simulink model "Test_algo_only"  (R2020b)
settings: Solver=ode4  StartTime=0.0  StopTime=0.05  FixedStep=0.001  RelTol=1e-3
values from neighbouring files (symbols this model uses):
  FFT_LENGTH = 256    [Init.m]
  Sampling_rate = 256e3    (= 256000)    [Init.m]
undefined symbols (not defined in the file or in its folder): InvMp, RotX
settings Model: Creator=franc  LastModifiedBy=franc

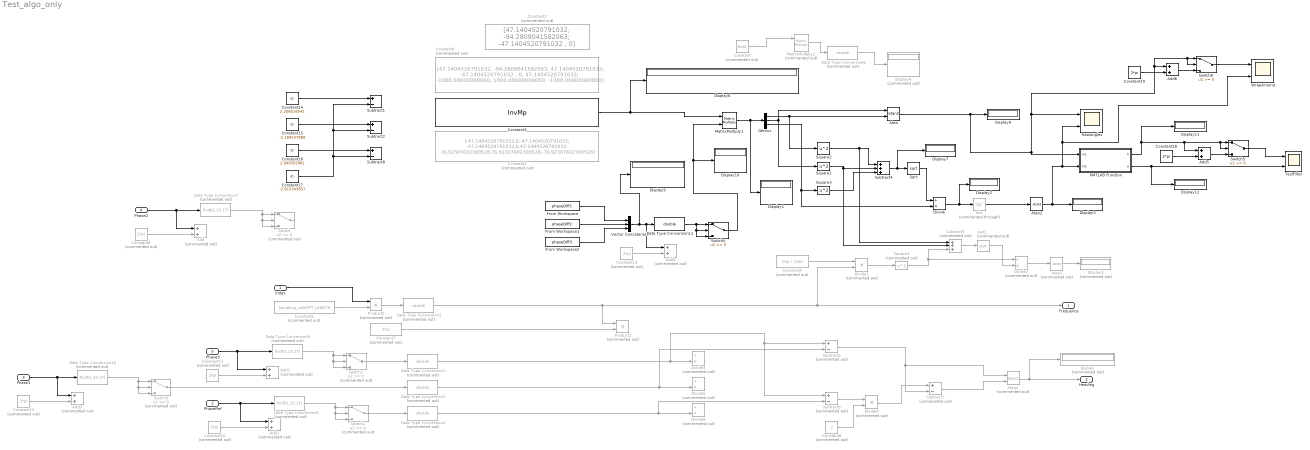
== system Test_algo_only ==
  Index : Inport
  PhaseRef : Inport  Port=2
  Phase1 : Inport  Port=3
  Phase2 : Inport  Port=4
  Phase3 : Inport  Port=5
  Abs : Abs  Commented=through
  Add{,1..4} (5 alike) : Sum  Commented=on
  Add5 : Sum
  Add6 : Sum
  Atan : Trigonometry  Operator=atan2  ApproximationMethod=CORDIC  OutputSignalType=real
  Atan1 : Trigonometry  Commented=on  Operator=acos  ApproximationMethod=CORDIC  OutputSignalType=real
  Atan2 : Trigonometry  Operator=acos  ApproximationMethod=CORDIC  OutputSignalType=real
  Atan4 : Trigonometry  Commented=on  Operator=atan2  ApproximationMethod=CORDIC  OutputSignalType=real
  Constant : Constant  Commented=on  Value=RotX
  Constant1 : Constant  Commented=on  Value=|  VectorParams1D=off  OutDataTypeStr=fixdt(1,15,7)
      | [-47.1404520791032,0,-47.1404520791032; -47.1404520791032,0,47.1404520791032;
      | -76.92307692300528,76.92307692300528,-76.92307692300528]
  Constant{9..13} (5 alike) : Constant  Commented=on  Value=2*pi  OutDataTypeStr=fixdt(0,16,12)  SampleTime=-1
  Constant14 : Constant  Value=2.206016541  OutDataTypeStr=double  SampleTime=-1
  Constant15 : Constant  Value=-2.184537888  OutDataTypeStr=double  SampleTime=-1
  Constant16 : Constant  Value=2.690505981  OutDataTypeStr=double  SampleTime=-1
  Constant17 : Constant  Value=-2.815343857  OutDataTypeStr=double  SampleTime=-1
  Constant18 : Constant  Value=2*pi  OutDataTypeStr=fixdt(0,16,12)  SampleTime=-1
  Constant19 : Constant  Value=2*pi  OutDataTypeStr=fixdt(0,16,12)  SampleTime=-1
  Constant2 : Constant  Commented=on  Value=|  VectorParams1D=off  OutDataTypeStr=fixdt(1,15,7)
      | [47.1404520791032,    -94.2809041582063;
      | -47.1404520791032 ,   0]
  Constant3 : Constant  Value=InvMp  VectorParams1D=off  OutDataTypeStr=fixdt(1,32,16)
  Constant4 : Constant  Commented=on  Value=2*pi / 1500
  Constant5 : Constant  Commented=on  Value=Sampling_rate/FFT_LENGTH  OutDataTypeStr=fixdt(0,10)  SampleTime=-1
  Constant6 : Constant  Commented=on  Value=|  VectorParams1D=off  OutDataTypeStr=fixdt(1,15,7)
      | [47.1404520791032,    -94.2809041582063,    47.1404520791032;
      | -47.1404520791032 ,   0,    47.1404520791032;
      | -1000.00000000000,   1000.00000000000,    -1000.00000000000]
  Constant7 : Constant  Commented=on  Value=2*pi  OutDataTypeStr=double
  Constant8 : Constant  Commented=on  Value=2  OutDataTypeStr=uint8
  Data Type Conversion{1..4,6} (5 alike) : DataTypeConversion  Commented=on  OutDataTypeStr=double
  Data Type Conversion{7..10} (4 alike) : DataTypeConversion  Commented=on  OutDataTypeStr=fixdt(1,23,17)
  Data Type Conversion11 : DataTypeConversion  OutDataTypeStr=double
  Demux : Demux  Outputs=3
  Display : Display  Commented=on
      settings: Decimation=8
  Display{1..3,6..12} (10 alike) : Display
  Display4 : Display  Commented=on
  Display5 : Display  Commented=on
  Divide : Product  Inputs=/*
  Divide1 : Product  Commented=on  Inputs=**  RndMeth=Zero  SaturateOnIntegerOverflow=on
  Divide2 : Product  Commented=on  Inputs=/*
  Divide3 : Product  Commented=on  Inputs=/*  RndMeth=Zero  SaturateOnIntegerOverflow=on
  Divide4 : Product  Commented=on  Inputs=**  RndMeth=Zero  SaturateOnIntegerOverflow=on
  Divide5 : Product  Commented=on  Inputs=/*  RndMeth=Zero  SaturateOnIntegerOverflow=on
  Divide6 : Product  Commented=on  Inputs=/*  RndMeth=Zero  SaturateOnIntegerOverflow=on
  From Workspace : FromWorkspace  VariableName=phaseDiff1  SampleTime=-1  Interpolate=off  OutputAfterFinalValue=Holding final value
  From Workspace1 : FromWorkspace  VariableName=phaseDiff2  SampleTime=-1  Interpolate=off  OutputAfterFinalValue=Holding final value
  From Workspace2 : FromWorkspace  VariableName=phaseDiff3  SampleTime=-1  Interpolate=off  OutputAfterFinalValue=Holding final value
  MATLAB Function : MATLAB Function  TreatAsAtomicUnit=on
  MatrixMultiply1 : Product  Multiplication=Matrix(*)
  MatrixMultiply2 : Product  Commented=on  Multiplication=Matrix(*)
  Product1 : Product  Commented=on
  Product2 : Product  Commented=on
  RawAngles : Scope  NumInputPorts=2
  Sqrt : Sqrt  OutDataTypeStr=double  SaturateOnIntegerOverflow=on
  Sqrt1 : Sqrt  Commented=on  OutDataTypeStr=double  SaturateOnIntegerOverflow=on
  Square1 : Math  Operator=square  SignedPower=on  RndMeth=Zero  SaturateOnIntegerOverflow=on  OutDataTypeStr=Inherit: Inherit via internal rule
  Square2 : Math  Operator=square  SignedPower=on  RndMeth=Zero  SaturateOnIntegerOverflow=on  OutDataTypeStr=Inherit: Inherit via internal rule
  Square3 : Math  Operator=square  SignedPower=on  RndMeth=Zero  SaturateOnIntegerOverflow=on  OutDataTypeStr=Inherit: Inherit via internal rule
  Square4 : Math  Commented=on  Operator=square  SignedPower=on  RndMeth=Zero  SaturateOnIntegerOverflow=on  OutDataTypeStr=Inherit: Inherit via internal rule
  Subtract1 : Sum  Inputs=+-
  Subtract2 : Sum  Inputs=+-
  Subtract3 : Sum  Commented=on  Inputs=+++
  Subtract4 : Sum  Inputs=+++
  Subtract5 : Sum  Commented=on  Inputs=+-
  Subtract6 : Sum  Commented=on  Inputs=+-
  Subtract7 : Sum  Commented=on  Inputs=+-
  Subtract8 : Sum  Inputs=+-
  Switch{,1..3} (4 alike) : Switch  Commented=on
  Switch4 : Switch
  Switch5 : Switch
  Switch6 : Switch
  TestFilter : Scope  NumInputPorts=2
  Vector Concatenate : Concatenate  NumInputs=3  Mode=Multidimensional array
  WrapAround : Scope  NumInputPorts=2
  Fréquence : Outport  InitialOutput=0
  Heading : Outport  Port=2  InitialOutput=0
  wires:
  MatrixMultiply1/1 -> Display1/1, Demux/1
  MatrixMultiply2/1 -> Data Type Conversion6/1
  Constant3/1 -> Display6/1, MatrixMultiply1/1
  Demux/2 -> Atan/1, Square1/1
  Constant/1 -> MatrixMultiply2/1
  Index/1 -> Product2/1
  Square1/1 -> Subtract3/2, Subtract4/2
  Square3/1 -> Subtract4/3
  Subtract4/1 -> Display7/1, Sqrt/1
  Demux/1 -> Square2/1, Atan/2
  Product2/1 -> Data Type Conversion2/1
  Constant11/1 -> Add2/2
  Switch3/1 -> Data Type Conversion3/1
  Phase3/1 -> Add2/1, Data Type Conversion9/1
  Constant9/1 -> Add/2
  Atan4/1 -> Display/1, Heading/1
  Atan1/1 -> Display5/1
  Switch2/1 -> Data Type Conversion1/1
  PhaseRef/1 -> Add1/1, Data Type Conversion8/1
  Square4/1 -> Divide2/1, Subtract3/3
  Data Type Conversion7/1 -> Switch/3, Switch/2, Switch/1
  Data Type Conversion10/1 -> Switch3/3, Switch3/2, Switch3/1
  Constant10/1 -> Add1/2
  Data Type Conversion3/1 -> Divide5/2, Subtract5/2
  Data Type Conversion9/1 -> Switch2/3, Switch2/2, Switch2/1
  Switch1/1 -> Data Type Conversion4/1
  Constant8/1 -> Divide4/2
  Constant7/1 -> Product1/2
  Data Type Conversion2/1 -> Product1/1, Divide1/2, Fréquence/1
  Constant4/1 -> Divide1/1
  Data Type Conversion4/1 -> Divide6/2, Subtract6/2
  Phase2/1 -> Add/1, Data Type Conversion7/1
  Square2/1 -> Subtract3/1, Subtract4/1
  Demux/3 -> Divide/2, Square3/1
  Subtract6/1 -> Divide4/1
  Subtract7/1 -> Atan4/2
  Divide2/1 -> Atan1/1
  Data Type Conversion6/1 -> Display4/1
  Divide1/1 -> Square4/1
  Sqrt1/1 -> Divide2/2
  Switch4/1 -> Display10/1, MatrixMultiply1/2
  Constant5/1 -> Product2/2
  Subtract5/1 -> Atan4/1, Subtract7/2
  Constant13/1 -> Add4/2
  Data Type Conversion8/1 -> Switch1/3, Switch1/2, Switch1/1
  Divide4/1 -> Subtract7/1
  Sqrt/1 -> Divide/1
  Constant12/1 -> Add3/2
  Phase1/1 -> Add3/1, Data Type Conversion10/1
  Data Type Conversion11/1 -> Switch4/3, Switch4/2, Switch4/1
  Data Type Conversion1/1 -> Divide3/2, Subtract6/1, Subtract5/1
  Subtract3/1 -> Sqrt1/1
  Vector Concatenate/1 -> Display9/1, Add4/1, Data Type Conversion11/1
  Constant16/1 -> Subtract8/1
  Constant15/1 -> Subtract2/1
  Constant14/1 -> Subtract1/1
  Constant17/1 -> Subtract8/2, Subtract1/2, Subtract2/2
  From Workspace1/1 -> Vector Concatenate/2
  From Workspace/1 -> Vector Concatenate/1
  From Workspace2/1 -> Vector Concatenate/3
  Atan/1 -> Switch6/2, Switch6/1, Add6/1, RawAngles/1, MATLAB Function/1(in1), Display8/1
  Divide/1 -> Abs/1, Display2/1
  Atan2/1 -> MATLAB Function/2(in2), RawAngles/2, WrapAround/2, Display3/1
  MATLAB Function/1(h) -> Add5/1, Switch5/2, Switch5/1, Display11/1
  MATLAB Function/2(e) -> Display12/1, TestFilter/2
  Abs/1 -> Atan2/1
  Constant18/1 -> Add5/2
  Add5/1 -> Switch5/3
  Switch5/1 -> TestFilter/1
  Constant19/1 -> Add6/2
  Add6/1 -> Switch6/3
  Switch6/1 -> WrapAround/1

== matlab function Test_algo_only/MATLAB Function ==
  data: in1 input; h output; in2 input; e output
function [h, e] = fcn(in1, in2)
    
    if in2 > pi/2
        e = pi - in2;
        if in1 < 0
            h = in1 + pi;
        else
            h = in1 - pi;
        end
    else
        h = in1;
        e = in2;
    end
end
